simulink model "Sensor_Data"  (R2021b)
settings: Solver=FixedStepDiscrete  StartTime=0.0  StopTime=10.0  RelTol=1e-3
undefined symbols (not defined in the file or in its folder): driving
libraries: drivingscenarioandsensors x4
(part 1 of 3)
settings Model: Creator=Admin  LastModifiedBy=Admin

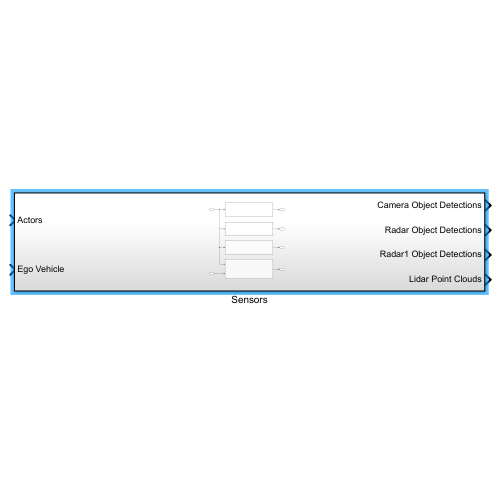
[thumbnail: Simulink's stored preview of the top-level diagram]
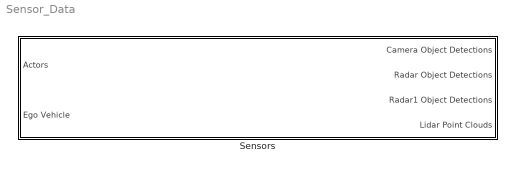
== system Sensor_Data ==
  Sensors : Subsystem
